simulink model "Linear_Moving_Setpoint_SS_PID"  (R2022a)
settings: Solver=VariableStepAuto  StartTime=tspan(1)  StopTime=tspan(2)  RelTol=1e-9
undefined symbols (not defined in the file): K1, K2, r_sim
libraries: cstblocks x4
settings Model: Creator=domin  LastModifiedBy=domin
settings SolverCC: AlgebraicLoopSolver=TrustRegion
settings DebuggingCC: AlgebraicLoopMsg=none  UnconnectedInputMsg=warning  UnconnectedOutputMsg=warning  UnconnectedLineMsg=warning  SFMachineParentedDataDiag=warning
settings RTWCC: DLArmComputeVersion=19.05

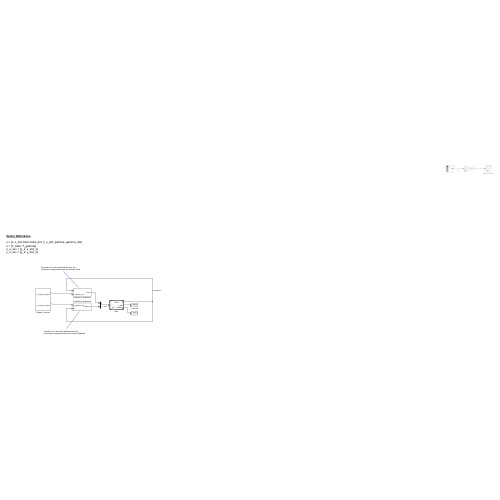
[thumbnail: Simulink's stored preview of the top-level diagram]
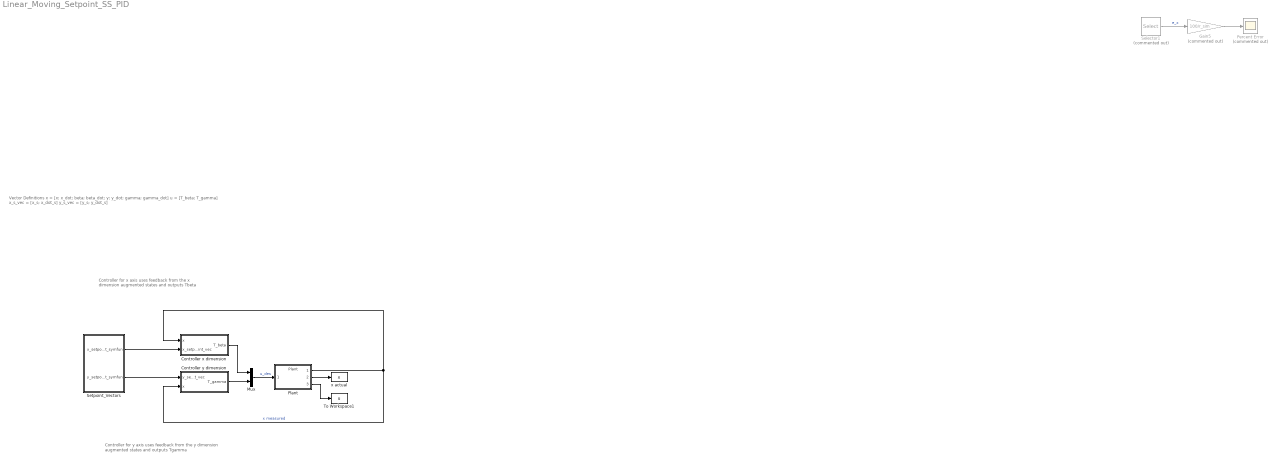
== system Linear_Moving_Setpoint_SS_PID ==
  note: Controller for y axis uses feedback from the
      | y dimension augmented states and outputs Tgamma
  note: Vector Definitions
      |
      | x = [x; x_dot; beta; beta_dot; y; y_dot; gamma; gamma_dot]
      | u = [T_beta; T_gamma]
      | x_s_vec = [x_s; x_dot_s]
      | y_s_vec = [y_s; y_dot_s]
  note: Controller for x axis uses feedback from the
      | x dimension augmented states and outputs Tbeta
  Controller x dimension : Subsystem
  Controller y dimension : Subsystem
  Gain5 : Gain  Commented=on  Gain=100/r_sim
  Mux : Mux  Inputs=2
  Percent Error : Scope  Commented=on
  Plant : ModelReference  ModelNameDialog=Plant  SimulationMode=Normal  ModelReferenceVersion=1.109
  Selector1 : Selector  Commented=on  InputPortWidth=5  IndexOptions=Index vector (dialog)  Indices=[1]  OutputSizes=1
  Setpoint_Vectors : Subsystem
  To Workspace1 : ToWorkspace  VariableName=u  SampleTime=-1
  x actual : ToWorkspace  VariableName=x  SampleTime=-1
  wires:
  Gain5/1 -> Percent Error/1
  Selector1/1 -> Gain5/1  "e_x"
  Controller x dimension/1(T_beta) -> Mux/1
  Controller y dimension/1(T_gamma) -> Mux/2
  Mux/1 -> Plant/1  "u_des"
  Plant/1 -> Controller x dimension/1(x), Controller y dimension/2(x)  "x measured"
  Plant/3 -> To Workspace1/1
  Plant/2 -> x actual/1
  Setpoint_Vectors/1(x_setpoint_symfun) -> Controller x dimension/2(x_setpoint_vec)
  Setpoint_Vectors/2(y_setpoint_symfun) -> Controller y dimension/1(y_setpoint_vec)

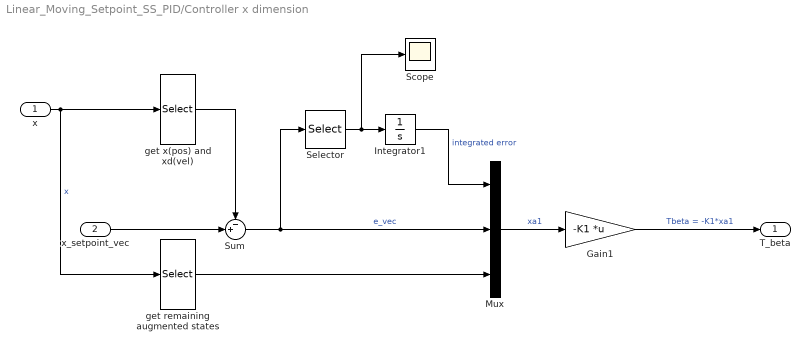
== system Linear_Moving_Setpoint_SS_PID/Controller x dimension ==
  x : Inport
  x_setpoint_vec : Inport  Port=2
  Gain1 : Gain  Gain=-K1  Multiplication=Matrix(K*u)
  Integrator1 : Integrator
  Mux : Mux  Inputs=3
  Scope : Scope
  Selector : Selector  InputPortWidth=2  IndexOptions=Index vector (dialog)  Indices=[1 ]  OutputSizes=1
  Sum : Sum  Inputs=-+|
  get remaining augmented states : Selector  InputPortWidth=8  IndexOptions=Index vector (dialog)  Indices=[3,4]  OutputSizes=1
  get x(pos) and xd(vel) : Selector  InputPortWidth=8  IndexOptions=Index vector (dialog)  Indices=[1 2]  OutputSizes=1
  T_beta : Outport
  wires:
  get remaining augmented states/1 -> Mux/3
  Gain1/1 -> T_beta/1  "Tbeta = -K1*xa1"
  get x(pos) and xd(vel)/1 -> Sum/1
  Mux/1 -> Gain1/1  "xa1"
  Sum/1 -> Selector/1, Mux/2  "e_vec"
  x_setpoint_vec/1 -> Sum/2
  x/1 -> get x(pos) and xd(vel)/1, get remaining augmented states/1  "x"
  Selector/1 -> Scope/1, Integrator1/1
  Integrator1/1 -> Mux/1  "integrated error"

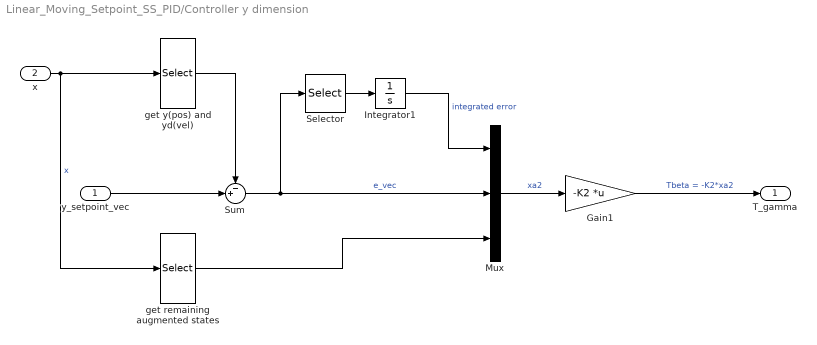
== system Linear_Moving_Setpoint_SS_PID/Controller y dimension ==
  y_setpoint_vec : Inport
  x : Inport  Port=2
  Gain1 : Gain  Gain=-K2  Multiplication=Matrix(K*u)
  Integrator1 : Integrator
  Mux : Mux  Inputs=3
  Selector : Selector  InputPortWidth=2  IndexOptions=Index vector (dialog)  Indices=[1 ]  OutputSizes=1
  Sum : Sum  Inputs=-+|
  get remaining augmented states : Selector  InputPortWidth=8  IndexOptions=Index vector (dialog)  Indices=[7,8]  OutputSizes=1
  get y(pos) and yd(vel) : Selector  InputPortWidth=8  IndexOptions=Index vector (dialog)  Indices=[5 6]  OutputSizes=1
  T_gamma : Outport
  wires:
  Integrator1/1 -> Mux/1  "integrated error"
  x/1 -> get y(pos) and yd(vel)/1, get remaining augmented states/1  "x"
  Gain1/1 -> T_gamma/1  "Tbeta = -K2*xa2"
  get y(pos) and yd(vel)/1 -> Sum/1
  Mux/1 -> Gain1/1  "xa2"
  get remaining augmented states/1 -> Mux/3
  Selector/1 -> Integrator1/1
  Sum/1 -> Selector/1, Mux/2  "e_vec"
  y_setpoint_vec/1 -> Sum/2

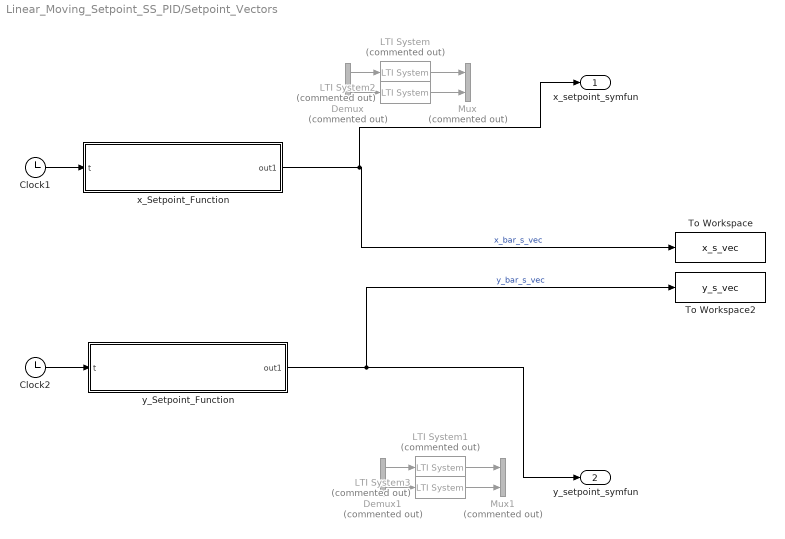
== system Linear_Moving_Setpoint_SS_PID/Setpoint_Vectors ==
  Clock1 : Clock
  Clock2 : Clock
  Demux : Demux  Commented=on  Outputs=2
  Demux1 : Demux  Commented=on  Outputs=2
  LTI System : cstblocks/LTI System  Commented=on  sys=x_s_tf  IC=[]
  LTI System1 : cstblocks/LTI System  Commented=on  sys=y_s_tf  IC=[]
  LTI System2 : cstblocks/LTI System  Commented=on  sys=x_s_tf  IC=[]
  LTI System3 : cstblocks/LTI System  Commented=on  sys=y_s_tf  IC=[]
  Mux : Mux  Commented=on  Inputs=2
  Mux1 : Mux  Commented=on  Inputs=2
  To Workspace : ToWorkspace  VariableName=x_s_vec  SampleTime=-1
  To Workspace2 : ToWorkspace  VariableName=y_s_vec  SampleTime=-1
  x_Setpoint_Function : MATLAB Function  TreatAsAtomicUnit=on
  y_Setpoint_Function : MATLAB Function  TreatAsAtomicUnit=on
  x_setpoint_symfun : Outport
  y_setpoint_symfun : Outport  Port=2
  wires:
  Clock2/1 -> y_Setpoint_Function/1(t)
  y_Setpoint_Function/1(out1) -> y_setpoint_symfun/1, To Workspace2/1  "y_bar_s_vec"
  Clock1/1 -> x_Setpoint_Function/1(t)
  LTI System/1 -> Mux/1
  x_Setpoint_Function/1(out1) -> x_setpoint_symfun/1, To Workspace/1  "x_bar_s_vec"
  Demux/2 -> LTI System2/1
  Demux/1 -> LTI System/1
  LTI System2/1 -> Mux/2
  LTI System3/1 -> Mux1/2
  Demux1/1 -> LTI System1/1
  Demux1/2 -> LTI System3/1
  LTI System1/1 -> Mux1/1

== matlab function Linear_Moving_Setpoint_SS_PID/Setpoint_Vectors/y_Setpoint_Function ==
  data: t input; out1 output
function out1 = y_s_vec(t)
%#codegen

%    This function was generated by the Symbolic Math Toolbox version 9.1.
%    18-Apr-2022 23:27:02

t2 = t./2.0;
t3 = (t.*pi)./3.0;
t4 = t.*pi.*(2.0./3.0);
t5 = -t2;
t7 = cos(t4);
t8 = sin(t3);
t6 = exp(t5);
t9 = t6-1.0;
out1 = [t7.*t8.*t9.*(-3.0./1.0e+1);t9.*((t8.*pi.*sin(t4))./5.0-(t7.*pi.*cos(t3))./1.0e+1)];

== matlab function Linear_Moving_Setpoint_SS_PID/Setpoint_Vectors/x_Setpoint_Function ==
  data: t input; out1 output
function out1 = x_s_vec(t)
%#codegen

%    This function was generated by the Symbolic Math Toolbox version 9.1.
%    18-Apr-2022 23:27:02

t2 = t./2.0;
t3 = (t.*pi)./3.0;
t4 = t.*pi.*(2.0./3.0);
t5 = -t2;
t7 = cos(t3);
t8 = cos(t4);
t6 = exp(t5);
t9 = t6-1.0;
out1 = [t7.*t8.*t9.*(-3.0./1.0e+1);t9.*((t7.*pi.*sin(t4))./5.0+(t8.*pi.*sin(t3))./1.0e+1)];
